simulink model "simulink_part2"  (R2021b)
settings: Solver=VariableStepAuto  StartTime=0.0  StopTime=10.0  RelTol=1e-3
values from neighbouring files (symbols this model uses):
  b = 3.5077e-06    [workspace_part2.mat]
  J = 3.2284e-05    [workspace_part2.mat]
  K = 0.0274    [workspace_part2.mat]
  L = 2.75e-06    [workspace_part2.mat]
  R = 4    [workspace_part2.mat]
settings Model: Creator=mahya  LastModifiedBy=hp

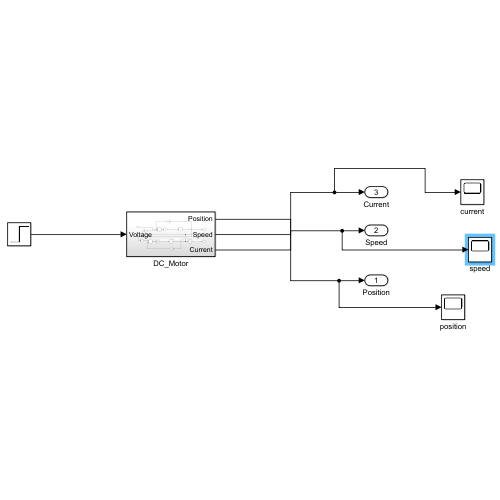
[thumbnail: Simulink's stored preview of the top-level diagram]
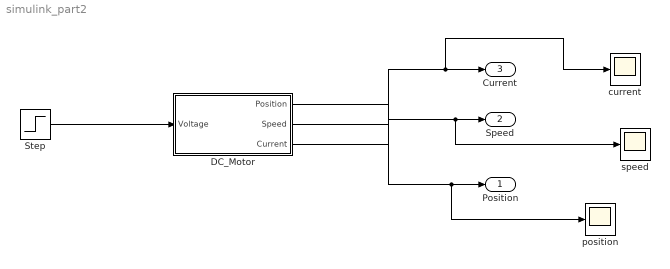
== system simulink_part2 ==
  DC_Motor : Subsystem
  Step : Step  Before=1  SampleTime=0
  current : Scope
  position : Scope
  speed : Scope
  Position : Outport
  Speed : Outport  Port=2
  Current : Outport  Port=3
  wires:
  Step/1 -> DC_Motor/1(Voltage)
  DC_Motor/1(Position) -> position/1, Position/1
  DC_Motor/2(Speed) -> speed/1, Speed/1
  DC_Motor/3(Current) -> current/1, Current/1

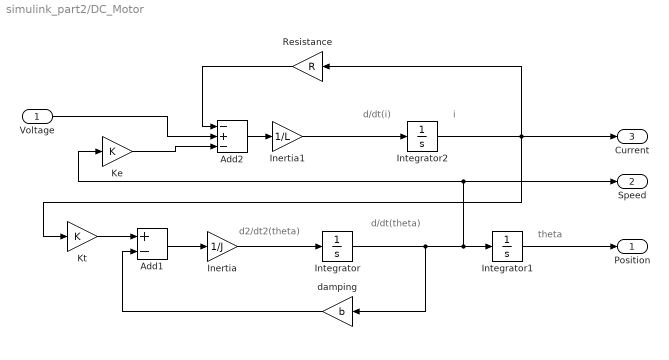
== system simulink_part2/DC_Motor ==
  note: d/dt(theta)
  note: d2/dt2(theta)
  note: theta
  note: d/dt(i)
  note: i
  Voltage : Inport
  Add1 : Sum  Inputs=+-
  Add2 : Sum  Inputs=-+-
  Inertia : Gain  Gain=1/J
  Inertia1 : Gain  Gain=1/L
  Integrator : Integrator  ContinuousStateAttributes='Integrator'
  Integrator1 : Integrator  ContinuousStateAttributes='Integrator1'
  Integrator2 : Integrator  ContinuousStateAttributes='Integrator1'
  Ke : Gain  Gain=K
  Kt : Gain  Gain=K
  Resistance : Gain  Gain=R
  damping : Gain  Gain=b
  Position : Outport
  Speed : Outport  Port=2
  Current : Outport  Port=3
  wires:
  damping/1 -> Add1/2
  Integrator2/1 -> Kt/1, Current/1, Resistance/1
  Inertia1/1 -> Integrator2/1
  Integrator/1 -> damping/1, Speed/1, Ke/1, Integrator1/1
  Add1/1 -> Inertia/1
  Ke/1 -> Add2/3
  Inertia/1 -> Integrator/1
  Kt/1 -> Add1/1
  Integrator1/1 -> Position/1
  Add2/1 -> Inertia1/1
  Resistance/1 -> Add2/1
  Voltage/1 -> Add2/2
